simulink model "compenatedsystemDisturbance"  (R2021b)
settings: Solver=VariableStepAuto  StartTime=0.0  StopTime=10.0  RelTol=1e-3
libraries: dspsrcs4 x4
settings Model: Creator=Asus  LastModifiedBy=Matina Kaviani
settings SolverCC: AlgebraicLoopSolver=TrustRegion
settings DebuggingCC: SFMachineParentedDataDiag=warning

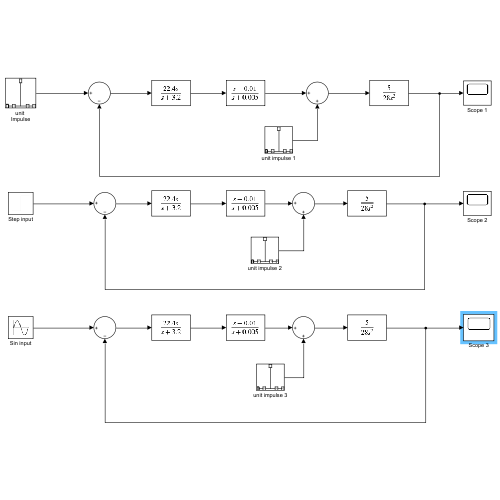
[thumbnail: Simulink's stored preview of the top-level diagram]
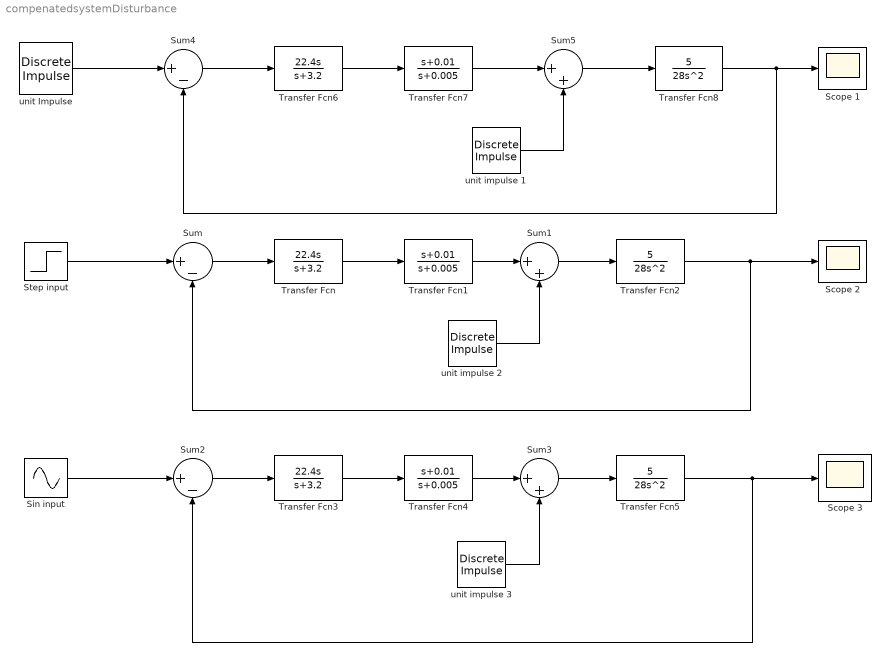
== system compenatedsystemDisturbance ==
  Scope 1 : Scope
  Scope 2 : Scope
  Scope 3 : Scope
  Sin input : Sin  Frequency=2*pi  SampleTime=0
  Step input : Step  After=2  SampleTime=0
  Sum : Sum  Inputs=|+-
  Sum1 : Sum  Inputs=|++
  Sum2 : Sum  Inputs=|+-
  Sum3 : Sum  Inputs=|++
  Sum4 : Sum  Inputs=|+-
  Sum5 : Sum  Inputs=|++
  Transfer Fcn : TransferFcn  Numerator=[22.4 0]  Denominator=[1 3.2]
  Transfer Fcn1 : TransferFcn  Numerator=[1 0.01]  Denominator=[1 0.005]
  Transfer Fcn2 : TransferFcn  Numerator=[0 5]  Denominator=[28 0 0]
  Transfer Fcn3 : TransferFcn  Numerator=[22.4 0]  Denominator=[1 3.2]
  Transfer Fcn4 : TransferFcn  Numerator=[1 0.01]  Denominator=[1 0.005]
  Transfer Fcn5 : TransferFcn  Numerator=[0 5]  Denominator=[28 0 0]
  Transfer Fcn6 : TransferFcn  Numerator=[22.4 0]  Denominator=[1 3.2]
  Transfer Fcn7 : TransferFcn  Numerator=[1 0.01]  Denominator=[1 0.005]
  Transfer Fcn8 : TransferFcn  Numerator=[0 5]  Denominator=[28 0 0]
  unit Impulse : dspsrcs4/Discrete  Impulse  Delay=0  SampleTime=1  FrameSample=1  OutputFrames=off  dataType=double  isSigned=on  wordLen=16  udDataType=sfix(16)  fracBitsMode=Best precision  numFracBits=15  OutDataTypeStr=double  LastOutDataTypeStr=double
  unit impulse 1 : dspsrcs4/Discrete  Impulse  Delay=0  SampleTime=1  FrameSample=1  OutputFrames=off  dataType=double  isSigned=on  wordLen=16  udDataType=sfix(16)  fracBitsMode=Best precision  numFracBits=15  OutDataTypeStr=double  LastOutDataTypeStr=double
  unit impulse 2 : dspsrcs4/Discrete  Impulse  Delay=0  SampleTime=1  FrameSample=1  OutputFrames=off  dataType=double  isSigned=on  wordLen=16  udDataType=sfix(16)  fracBitsMode=Best precision  numFracBits=15  OutDataTypeStr=double  LastOutDataTypeStr=double
  unit impulse 3 : dspsrcs4/Discrete  Impulse  Delay=0  SampleTime=1  FrameSample=1  OutputFrames=off  dataType=double  isSigned=on  wordLen=16  udDataType=sfix(16)  fracBitsMode=Best precision  numFracBits=15  OutDataTypeStr=double  LastOutDataTypeStr=double
  wires:
  Step input/1 -> Sum/1
  Sin input/1 -> Sum2/1
  Sum/1 -> Transfer Fcn/1
  Transfer Fcn/1 -> Transfer Fcn1/1
  Transfer Fcn1/1 -> Sum1/1
  Sum1/1 -> Transfer Fcn2/1
  Transfer Fcn2/1 -> Sum/2, Scope 2/1
  unit impulse 2/1 -> Sum1/2
  Sum2/1 -> Transfer Fcn3/1
  Transfer Fcn3/1 -> Transfer Fcn4/1
  Transfer Fcn4/1 -> Sum3/1
  unit impulse 3/1 -> Sum3/2
  Sum3/1 -> Transfer Fcn5/1
  Transfer Fcn5/1 -> Sum2/2, Scope 3/1
  unit Impulse/1 -> Sum4/1
  Sum4/1 -> Transfer Fcn6/1
  Transfer Fcn6/1 -> Transfer Fcn7/1
  Transfer Fcn7/1 -> Sum5/1
  Sum5/1 -> Transfer Fcn8/1
  Transfer Fcn8/1 -> Sum4/2, Scope 1/1
  unit impulse 1/1 -> Sum5/2
